simulink model "hw4_sim"  (R2018b)
settings: Solver=FixedStepAuto  StartTime=0.0  StopTime=stopTime  FixedStep=1/60  RelTol=1e-3
values from neighbouring files (symbols this model uses):
  B = 0    [hw4.m]    (also in hw4_main.m; hw4_q1.m; hw4_q2.m = 0.1; hw4_q3.m)
  g = 9.8    [hw4.m]    (also in hw4_main.m; hw4_q1.m; hw4_q2.m; hw4_q3.m)
  K1 = 20    [hw4.m]    (also in hw4_main.m; hw4_q1.m; hw4_q2.m; hw4_q3.m)
  L = L1 + L2    (= 0.5)    [hw4.m]    (also in hw4_main.m; hw4_q1.m; hw4_q2.m; hw4_q3.m)
  L1 = 0.25    [hw4.m]    (also in hw4_main.m; hw4_q1.m; hw4_q2.m; hw4_q3.m)
  M1 = 10    [hw4.m]    (also in hw4_main.m; hw4_q1.m; hw4_q2.m; hw4_q3.m)
  M2 = 10    [hw4.m]    (also in hw4_main.m; hw4_q1.m; hw4_q2.m; hw4_q3.m)
  stepInputTime = 3    [hw4.m]    (also in hw4_main.m; hw4_q1.m; hw4_q2.m; hw4_q3.m)
  tau1_final = 0    [hw4.m]    (also in hw4_main.m; hw4_q1.m; hw4_q2.m; hw4_q3.m)
  tau1_init = 35    [hw4.m]    (also in hw4_main.m = M1*g*L*sin(theta1_init); hw4_q1.m = M1*g*L*sin(theta1_init); hw4_q2.m; hw4_q3.m)
  tau2_final = 0    [hw4.m]    (also in hw4_main.m; hw4_q1.m; hw4_q2.m; hw4_q3.m)
  tau2_init = 25    [hw4.m]    (also in hw4_main.m = M2*g*L*sin(theta2_init); hw4_q1.m = M2*g*L*sin(theta2_init); hw4_q2.m; hw4_q3.m)
  theta1_init = 45 * pi / 180    (= 0.785398163397)    [hw4.m]    (also in hw4_main.m; hw4_q1.m; hw4_q2.m; hw4_q3.m)
  theta2_init = 30 * pi / 180    (= 0.523598775598)    [hw4.m]    (also in hw4_main.m; hw4_q1.m; hw4_q2.m; hw4_q3.m = 0.785398163397)
settings Model: Creator=CHENG  LastModifiedBy=CHENG

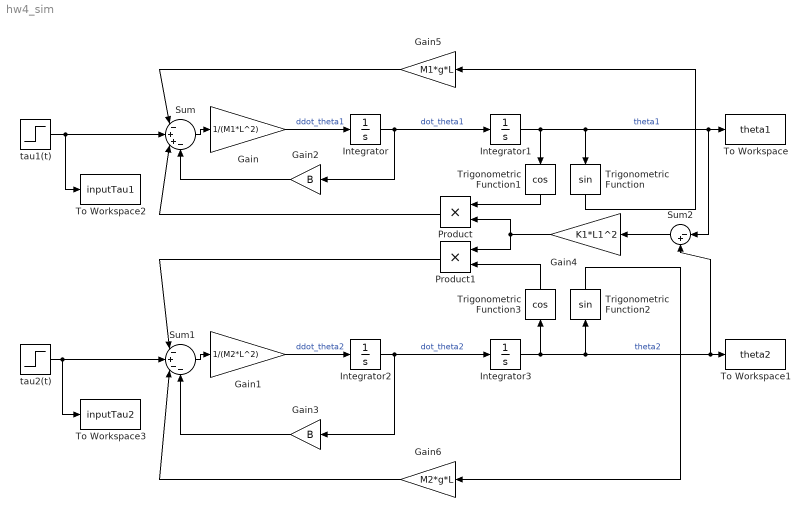
== system hw4_sim ==
  Gain : Gain  Gain=1/(M1*L^2)
  Gain1 : Gain  Gain=1/(M2*L^2)
  Gain2 : Gain  Gain=B
  Gain3 : Gain  Gain=B
  Gain4 : Gain  Gain=K1*L1^2
  Gain5 : Gain  Gain=M1*g*L
  Gain6 : Gain  Gain=M2*g*L
  Integrator : Integrator
  Integrator1 : Integrator  InitialCondition=theta1_init
  Integrator2 : Integrator
  Integrator3 : Integrator  InitialCondition=theta2_init
  Product : Product
  Product1 : Product
  Sum : Sum  Inputs=|-++-
  Sum1 : Sum  Inputs=|-+--
  Sum2 : Sum  Inputs=|-+
  To Workspace : ToWorkspace  VariableName=theta1  SaveFormat=Timeseries  SampleTime=-1
  To Workspace1 : ToWorkspace  VariableName=theta2  SaveFormat=Timeseries  SampleTime=-1
  To Workspace2 : ToWorkspace  VariableName=inputTau1  SaveFormat=Timeseries  SampleTime=-1
  To Workspace3 : ToWorkspace  VariableName=inputTau2  SaveFormat=Timeseries  SampleTime=-1
  Trigonometric Function : Trigonometry
  Trigonometric Function1 : Trigonometry  Operator=cos
  Trigonometric Function2 : Trigonometry
  Trigonometric Function3 : Trigonometry  Operator=cos
  tau1(t) : Step  Time=stepInputTime  Before=tau1_init  After=tau1_final  SampleTime=0
  tau2(t) : Step  Time=stepInputTime  Before=tau2_init  After=tau2_final  SampleTime=0
  wires:
  Integrator/1 -> Gain2/1, Integrator1/1  "dot_theta1"
  Gain/1 -> Integrator/1  "ddot_theta1"
  Sum/1 -> Gain/1
  Integrator1/1 -> Trigonometric Function1/1, Trigonometric Function/1, Sum2/1, To Workspace/1  "theta1"
  Integrator3/1 -> Trigonometric Function3/1, Trigonometric Function2/1, To Workspace1/1, Sum2/2  "theta2"
  Sum1/1 -> Gain1/1
  tau2(t)/1 -> To Workspace3/1, Sum1/2
  Gain1/1 -> Integrator2/1  "ddot_theta2"
  Integrator2/1 -> Gain3/1, Integrator3/1  "dot_theta2"
  Gain2/1 -> Sum/4
  Gain3/1 -> Sum1/4
  Trigonometric Function/1 -> Gain5/1
  Sum2/1 -> Gain4/1
  Trigonometric Function3/1 -> Product1/2
  Trigonometric Function1/1 -> Product/1
  Gain4/1 -> Product/2, Product1/1
  Product/1 -> Sum/3
  tau1(t)/1 -> To Workspace2/1, Sum/2
  Gain5/1 -> Sum/1
  Trigonometric Function2/1 -> Gain6/1
  Gain6/1 -> Sum1/3
  Product1/1 -> Sum1/1
